simulink model "DCMotorSmlnk"  (Simulink 7.7)
settings: Solver=ode45  StartTime=0.0  StopTime=10  RelTol=1e-6
values from neighbouring files (symbols this model uses):
  A = DCMotor_cont.A    [DCMotor.m]
  B = DCMotor_cont.B    [DCMotor.m]
  C = eye(size(A))    [DCMotor.m]
  D = 0*B    (= 0)    [DCMotor.m]
  DCMotorController_name = 'DCMotorSWController2'    [DCMotor.m]
  uini = 0    [DCMotor.m]
  xini = [0;0]    [DCMotor.m]
settings Model: Creator=manuelmazo  LastModifiedBy=manuelmazo  ExtModeAutoUpdateStatusClock=off
settings OptimizationCC: InitFltsAndDblsToZero=on
settings DebuggingCC: SaveWithParameterizedLinksMsg=none  StrictBusMsg=Warning
settings SFSimCC: SimParseCustomCode=off
settings GRTTargetCC: TargetFcnLib=ansi_tfl_tmw.mat

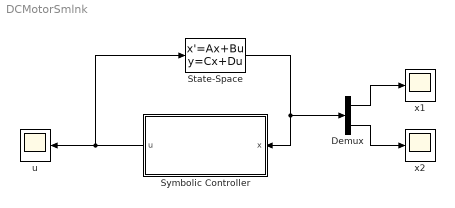
== system DCMotorSmlnk ==
  Demux : Demux  Outputs=2
  State-Space : StateSpace  A=A  B=B  C=C  D=D  X0=xini
  "Symbolic Controller " : Subsystem  mask{contr_name=DCMotorController_name, uini=uini}
      mask prompts: contr_name "Controller Name"; uini "Initial Controller State"
      mask init:
      | load(strcat(contr_name,'_symb'), 'params_symb');
  u : Scope
      settings: SaveName=ScopeData3
  x1 : Scope
  x2 : Scope
      settings: SaveName=ScopeData2
  wires:
  State-Space/1 -> Demux/1, "Symbolic Controller "/1(x)
  Demux/1 -> x1/1
  Demux/2 -> x2/1
  "Symbolic Controller "/1(u) -> State-Space/1, u/1

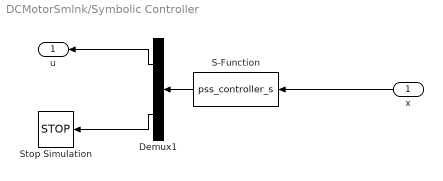
== system DCMotorSmlnk/Symbolic Controller  ==
  x : Inport
  Demux1 : Demux  Outputs=2
  S-Function : S-Function  FunctionName=pss_controller_s  Parameters=params_symb, contr_name, uini  EnableBusSupport=off
  Stop Simulation : Stop
  u : Outport
  wires:
  S-Function/1 -> Demux1/1
  x/1 -> S-Function/1
  Demux1/1 -> u/1
  Demux1/2 -> Stop Simulation/1
